simulink library "AR_Drone_Networking"  (R2016a)
settings: Solver=ode45  StartTime=0.0  StopTime=10.0  RelTol=1e-3
libraries: dspnetwork x1
settings Model: Creator=sannem  LastModifiedBy=sannem
settings DataIOCC: LimitDataPoints=on
settings DebuggingCC: AllowSymbolicDim=off

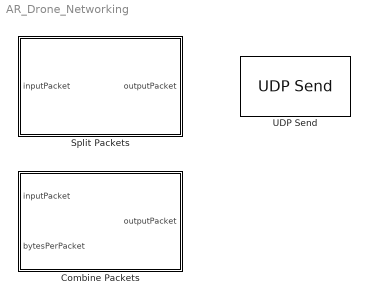
== system AR_Drone_Networking ==
  Combine Packets : MATLAB Function  TreatAsAtomicUnit=on  mask(AR Drone 2.0: Combine Packets){fullPacketSize=15000}
      mask prompts: fullPacketSize "Full packet size"
      mask help: This block will combine incombing packets of fixed size into packets of the user defined full packet size using header information inside the packets for reconstruction.
  Split Packets : MATLAB Function  TreatAsAtomicUnit=on  mask(AR Drone 2.0: Split Packets){bytesPerPacket=15000}
      mask prompts: bytesPerPacket "Bytes per packet"
      mask help: This block splits an input array into packages of user specified maximum packet size, including a single byte as a header.
  UDP Send : dspnetwork/UDP Send  remoteURL='192.168.1.2'  remotePort=24000  localURL='0.0.0.0'  localPortSource=Automatically determine  localPort=-1  sampletime=-1  blockPlatform=LINUX  separateLengthPort=0  mask(UDP Send){}

== matlab function AR_Drone_Networking/Combine Packets ==
  data: inputPacket input; outputPacket output; fullPacketSize parameter; bytesPerPacket input
function outputPacket  = CombinePackets(inputPacket, fullPacketSize, bytesPerPacket)

persistent tempOutputPacket     % packet where the incoming subpackets are written to
if isempty(tempOutputPacket)
    tempOutputPacket = zeros(1,fullPacketSize);
end

dataPerPacket = double(bytesPerPacket) - 1; % remove 1 byte for the header  
header = double(inputPacket(1));
startIndex = 1;
if header > 0
    startIndex = ((header - 1) * dataPerPacket) + 1;
end
endIndex = min(header * dataPerPacket, fullPacketSize);
tempOutputPacket(startIndex : endIndex) = uint8(inputPacket(2 : endIndex - startIndex + 2));
outputPacket = uint8(tempOutputPacket);
% outputPacket = uint8(zeros(1,fullPacketSize));

end

== matlab function AR_Drone_Networking/Split Packets ==
  data: inputPacket input; outputPacket output; bytesPerPacket parameter
function outputPacket = SplitPackets(inputPacket, bytesPerPacket)

dataPerPacket = bytesPerPacket - 1; % remove 1 byte for the header

persistent counter  % keeps track of how many sub packets have been send
if isempty(counter)
   counter = 1;
end

persistent packetInBuffer % storage of the whole packet to be send
if isempty(packetInBuffer)
    packetInBuffer = inputPacket;
end

subPacketCount = length(inputPacket) / dataPerPacket;   % compute how many packets are needed
if (floor(subPacketCount) ~= subPacketCount || subPacketCount == 0 )  
   subPacketCount = floor(subPacketCount) + 1;  % Make sure the packet count is a whole number > 0
end

packetLength = dataPerPacket;
if (counter * dataPerPacket > length(packetInBuffer)) % if the sub packet is smaller than bitsPerPacket, adjust the packet length
    packetLength = mod(length(packetInBuffer),dataPerPacket); 
end

startIndex = dataPerPacket * (counter - 1) + 1;
outputPacket = uint8(zeros(1, bytesPerPacket));
outputPacket(1,1) = uint8(counter);  % add a header
% outputPacket(1, 2 : packetLength + 1) =  uint8(inputPacket(startIndex : startIndex + packetLength ));
% Use a for loop to avoid variable signal size warning
for n = 2 : packetLength + 1;   
    outputPacket(1,n) = uint8(inputPacket(startIndex + n - 2));
end

counter = counter + 1;
if counter > subPacketCount
   counter = 1;
   packetInBuffer = inputPacket; %  Put a new input packet in the buffer
end

end
